simulink model "attitude_control"  (R2024b)
settings: Solver=FixedStepAuto  StartTime=0.0  StopTime=1000  FixedStep=1  RelTol=1e-3
values from neighbouring files (symbols this model uses):
  H0 = [30; 30; 30]    [initialcondition.m]
  I = [1759 0 0; 0 2758 0; 0 0 2171]    [initialcondition.m]
  kxd = 395.4913    [initialcondition.m]    (also in pd_fitness.m = x(4); pd_show.m = out.kxd)
  kxp = 18.1115    [initialcondition.m]    (also in pd_fitness.m = x(1); pd_show.m = out.kxp)
  kyd = 172.6452    [initialcondition.m]    (also in pd_fitness.m = x(5); pd_show.m = out.kyd)
  kyp = 7.3074    [initialcondition.m]    (also in pd_fitness.m = x(2); pd_show.m = out.kyp)
  kzd = 636.1855    [initialcondition.m]    (also in pd_fitness.m = x(6); pd_show.m = out.kzd)
  kzp = 21.1317    [initialcondition.m]    (also in pd_fitness.m = x(3); pd_show.m = out.kzp)
  qZYX = eul2quat(Euler0)    [initialcondition.m]
  w0 = [0; 0; 0]    [initialcondition.m]
settings Model: Creator=ThinkBook  LastModifiedBy=Lzy18
settings DebuggingCC: UnconnectedInputMsg=warning  UnconnectedOutputMsg=warning  UnconnectedLineMsg=warning
settings ModelReferenceCC: EnableRefExpFcnMdlSchedulingChecks=on
settings RTWCC: GPUComputeCapability=3.5  DLArmComputeVersion=19.05

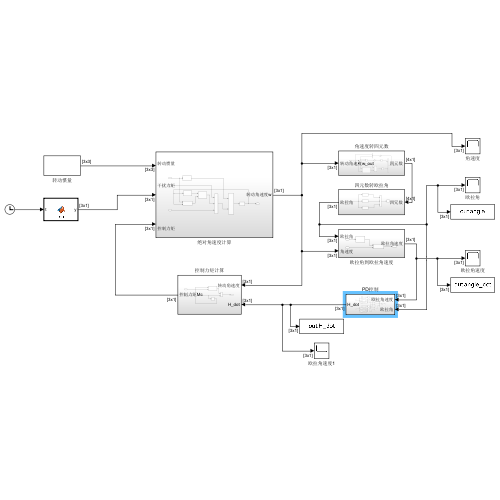
[thumbnail: Simulink's stored preview of the top-level diagram]
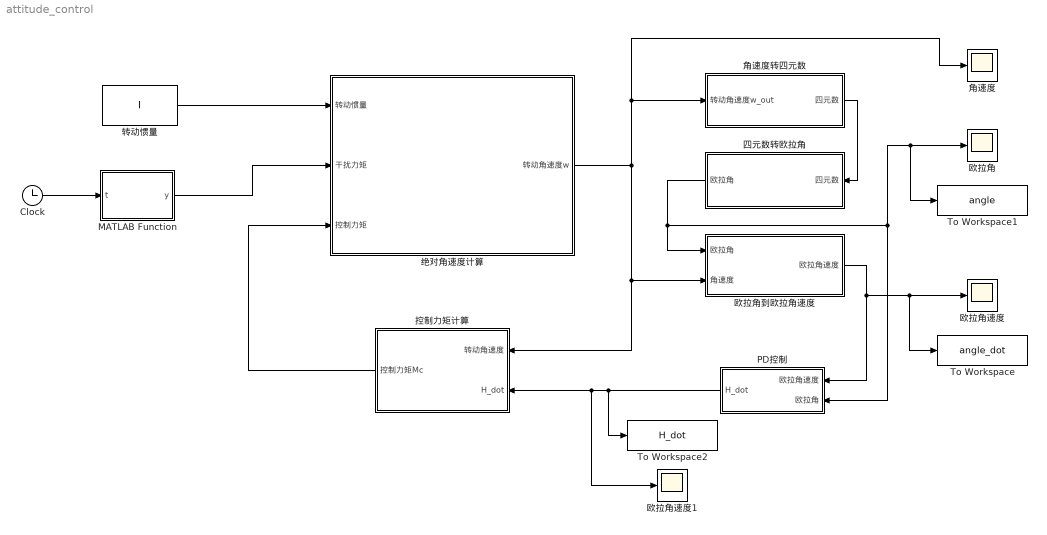
== system attitude_control ==
  Clock : Clock
  MATLAB Function : MATLAB Function  TreatAsAtomicUnit=on
  PD控制 : Subsystem
  To Workspace : ToWorkspace  VariableName=angle_dot  SampleTime=-1
  To Workspace1 : ToWorkspace  VariableName=angle  SampleTime=-1
  To Workspace2 : ToWorkspace  VariableName=H_dot  SampleTime=-1
  四元数转欧拉角 : Subsystem
  控制力矩计算 : Subsystem
  欧拉角 : Scope
  欧拉角到欧拉角速度 : Subsystem
  欧拉角速度 : Scope
  欧拉角速度1 : Scope
  绝对角速度计算 : Subsystem
  角速度 : Scope
  角速度转四元数 : Subsystem
  转动惯量 : Constant  Value=I
  wires:
  转动惯量/1 -> 绝对角速度计算/1(转动惯量)
  控制力矩计算/1(控制力矩Mc) -> 绝对角速度计算/3(控制力矩)
  绝对角速度计算/1(转动角速度w) -> 角速度/1, 角速度转四元数/1(转动角速度w_out), 控制力矩计算/1(转动角速度), 欧拉角到欧拉角速度/2(角速度)
  角速度转四元数/1(四元数) -> 四元数转欧拉角/1(四元数)
  PD控制/1(H_dot) -> To Workspace2/1, 欧拉角速度1/1, 控制力矩计算/2(H_dot)
  四元数转欧拉角/1(欧拉角) -> 欧拉角到欧拉角速度/1(欧拉角), PD控制/2(欧拉角), To Workspace1/1, 欧拉角/1
  MATLAB Function/1(y) -> 绝对角速度计算/2(干扰力矩)
  Clock/1 -> MATLAB Function/1(t)
  欧拉角到欧拉角速度/1(欧拉角速度) -> PD控制/1(欧拉角速度), To Workspace/1, 欧拉角速度/1

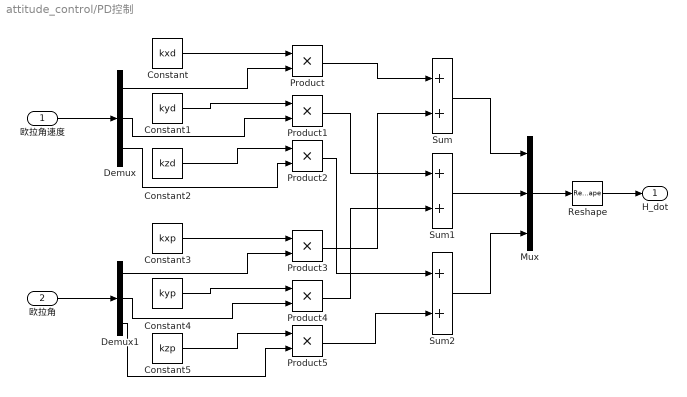
== system attitude_control/PD控制 ==
  欧拉角速度 : Inport
  欧拉角 : Inport  Port=2
  Constant : Constant  Value=kxd
  Constant1 : Constant  Value=kyd
  Constant2 : Constant  Value=kzd
  Constant3 : Constant  Value=kxp
  Constant4 : Constant  Value=kyp
  Constant5 : Constant  Value=kzp
  Demux : Demux  Outputs=3
  Demux1 : Demux  Outputs=3
  Mux : Mux  Inputs=3
  Product{,1..5} (6 alike) : Product
  Reshape : Reshape  OutputDimensionality=Customize  OutputDimensions=[3,1]
  Sum : Sum
  Sum1 : Sum
  Sum2 : Sum
  H_dot : Outport
  wires:
  欧拉角速度/1 -> Demux/1
  欧拉角/1 -> Demux1/1
  Demux/1 -> Product/2
  Constant/1 -> Product/1
  Constant1/1 -> Product1/1
  Demux/2 -> Product1/2
  Constant2/1 -> Product2/1
  Demux/3 -> Product2/2
  Constant5/1 -> Product5/1
  Constant3/1 -> Product3/1
  Demux1/1 -> Product3/2
  Constant4/1 -> Product4/1
  Demux1/2 -> Product4/2
  Demux1/3 -> Product5/2
  Product/1 -> Sum/1
  Product3/1 -> Sum/2
  Sum/1 -> Mux/1
  Sum1/1 -> Mux/2
  Sum2/1 -> Mux/3
  Product1/1 -> Sum1/1
  Product4/1 -> Sum1/2
  Product2/1 -> Sum2/1
  Product5/1 -> Sum2/2
  Mux/1 -> Reshape/1
  Reshape/1 -> H_dot/1

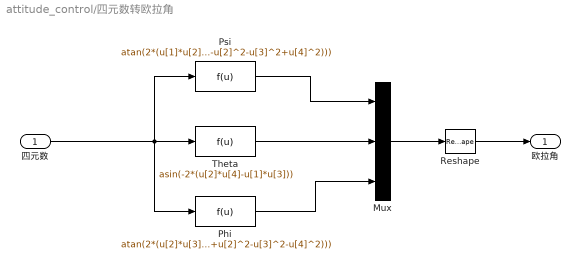
== system attitude_control/四元数转欧拉角 ==
  四元数 : Inport
  Mux : Mux  Inputs=3
  Phi : Fcn  Expr=atan(2*(u[2]*u[3]+u[1]*u[4]/(u[1]^2+u[2]^2-u[3]^2-u[4]^2)))
  Psi : Fcn  Expr=atan(2*(u[1]*u[2]+u[3]*u[4]/(u[1]^2-u[2]^2-u[3]^2+u[4]^2)))
  Reshape : Reshape  OutputDimensionality=Customize  OutputDimensions=[3,1]
  Theta : Fcn  Expr=asin(-2*(u[2]*u[4]-u[1]*u[3]))
  欧拉角 : Outport
  wires:
  Psi/1 -> Mux/1
  四元数/1 -> Phi/1, Psi/1, Theta/1
  Theta/1 -> Mux/2
  Phi/1 -> Mux/3
  Mux/1 -> Reshape/1
  Reshape/1 -> 欧拉角/1

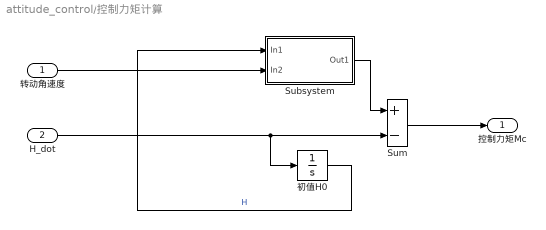
== system attitude_control/控制力矩计算 ==
  转动角速度 : Inport
  H_dot : Inport  Port=2
  Subsystem : Subsystem
      mask Display:
      | disp('Cross \nProduct')
      | port_label('input',1,'X')
      | port_label('input',2,'Y')
      | port_label('output',1,'X*Y')
  Sum : Sum  Inputs=+-
  初值H0 : Integrator  InitialCondition=H0
  控制力矩Mc : Outport
  wires:
  Sum/1 -> 控制力矩Mc/1
  转动角速度/1 -> Subsystem/2(In2)
  H_dot/1 -> Sum/2, 初值H0/1
  Subsystem/1(Out1) -> Sum/1
  初值H0/1 -> Subsystem/1(In1)  "H"

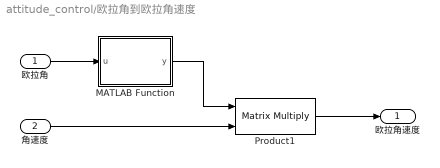
== system attitude_control/欧拉角到欧拉角速度 ==
  欧拉角 : Inport
  角速度 : Inport  Port=2
  MATLAB Function : MATLAB Function  TreatAsAtomicUnit=on
  Product1 : Product  Multiplication=Matrix(*)
  欧拉角速度 : Outport
  wires:
  Product1/1 -> 欧拉角速度/1
  欧拉角/1 -> MATLAB Function/1(u)
  MATLAB Function/1(y) -> Product1/1
  角速度/1 -> Product1/2

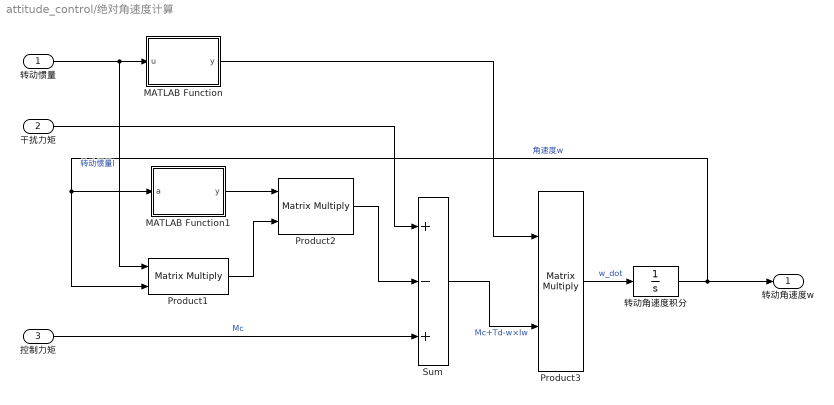
== system attitude_control/绝对角速度计算 ==
  转动惯量 : Inport
  干扰力矩 : Inport  Port=2
  控制力矩 : Inport  Port=3
  MATLAB Function : MATLAB Function  TreatAsAtomicUnit=on
  MATLAB Function1 : MATLAB Function  TreatAsAtomicUnit=on
  Product1 : Product  Multiplication=Matrix(*)
  Product2 : Product  Multiplication=Matrix(*)
  Product3 : Product  Multiplication=Matrix(*)
  Sum : Sum  Inputs=+-+
  转动角速度积分 : Integrator  InitialCondition=w0
  转动角速度w : Outport
  wires:
  Sum/1 -> Product3/2  "Mc+Td-w×Iw"
  Product3/1 -> 转动角速度积分/1  "w_dot"
  转动角速度积分/1 -> Product1/2, MATLAB Function1/1(a), 转动角速度w/1  "角速度w"
  转动惯量/1 -> MATLAB Function/1(u), Product1/1  "转动惯量I"
  控制力矩/1 -> Sum/3  "Mc"
  MATLAB Function/1(y) -> Product3/1
  MATLAB Function1/1(y) -> Product2/1
  Product1/1 -> Product2/2
  Product2/1 -> Sum/2
  干扰力矩/1 -> Sum/1

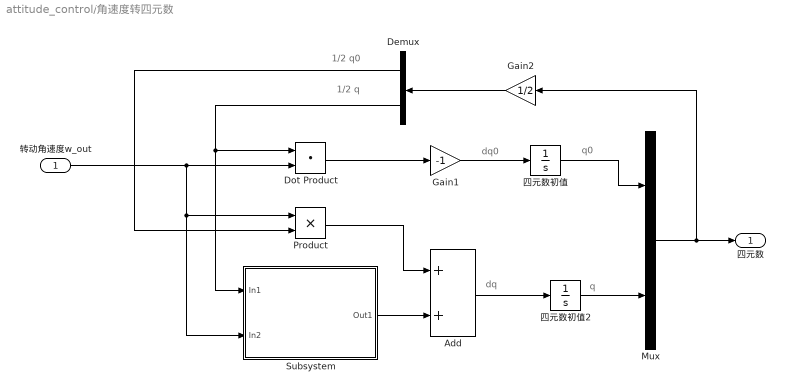
== system attitude_control/角速度转四元数 ==
  note: q
  note: dq
  note: dq0
  note: q0
  note: 1/2 q0
  note: 1/2 q
  转动角速度w_out : Inport
  Add : Sum
  Demux : Demux  Outputs=2
  Dot Product : DotProduct  OutDataTypeStr=Inherit: Inherit via internal rule
  Gain1 : Gain  Gain=-1
  Gain2 : Gain  Gain=1/2
  Mux : Mux  Inputs=[1 3]
  Product : Product
  Subsystem : Subsystem
      mask Display:
      | disp('Cross \nProduct')
      | port_label('input',1,'X')
      | port_label('input',2,'Y')
      | port_label('output',1,'X*Y')
  四元数初值 : Integrator  InitialCondition=qZYX(1)
  四元数初值2 : Integrator  InitialCondition=qZYX(2:4)'
  四元数 : Outport
  wires:
  Demux/2 -> Dot Product/1, Subsystem/1(In1)
  Gain1/1 -> 四元数初值/1
  Subsystem/1(Out1) -> Add/2
  四元数初值/1 -> Mux/1
  Demux/1 -> Product/2
  Gain2/1 -> Demux/1
  Mux/1 -> Gain2/1, 四元数/1
  转动角速度w_out/1 -> Product/1, Subsystem/2(In2), Dot Product/2
  Add/1 -> 四元数初值2/1
  Dot Product/1 -> Gain1/1
  四元数初值2/1 -> Mux/2
  Product/1 -> Add/1

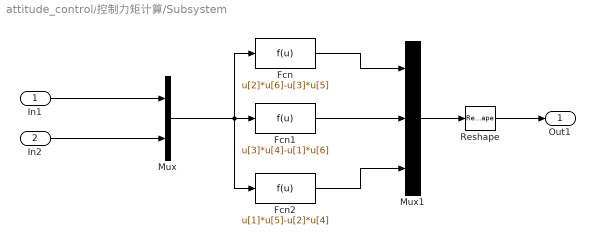
== system attitude_control/控制力矩计算/Subsystem ==
  In1 : Inport
  In2 : Inport  Port=2
  Fcn : Fcn  Expr=u[2]*u[6]-u[3]*u[5]
  Fcn1 : Fcn  Expr=u[3]*u[4]-u[1]*u[6]
  Fcn2 : Fcn  Expr=u[1]*u[5]-u[2]*u[4]
  Mux : Mux  Inputs=2
  Mux1 : Mux  Inputs=3
  Reshape : Reshape  OutputDimensionality=Customize  OutputDimensions=[3,1]
  Out1 : Outport
  wires:
  In2/1 -> Mux/2
  In1/1 -> Mux/1
  Fcn/1 -> Mux1/1
  Fcn1/1 -> Mux1/2
  Fcn2/1 -> Mux1/3
  Mux/1 -> Fcn2/1, Fcn/1, Fcn1/1
  Reshape/1 -> Out1/1
  Mux1/1 -> Reshape/1

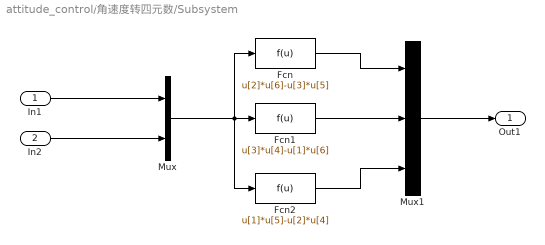
== system attitude_control/角速度转四元数/Subsystem ==
  In1 : Inport
  In2 : Inport  Port=2
  Fcn : Fcn  Expr=u[2]*u[6]-u[3]*u[5]
  Fcn1 : Fcn  Expr=u[3]*u[4]-u[1]*u[6]
  Fcn2 : Fcn  Expr=u[1]*u[5]-u[2]*u[4]
  Mux : Mux  Inputs=2
  Mux1 : Mux  Inputs=3
  Out1 : Outport
  wires:
  In2/1 -> Mux/2
  In1/1 -> Mux/1
  Fcn/1 -> Mux1/1
  Fcn1/1 -> Mux1/2
  Fcn2/1 -> Mux1/3
  Mux/1 -> Fcn2/1, Fcn/1, Fcn1/1
  Mux1/1 -> Out1/1

== matlab function attitude_control/绝对角速度计算/MATLAB Function ==
  data: u input; y output
function y = fcn(u)

y = inv(u);

end

== matlab function attitude_control/绝对角速度计算/MATLAB Function1 ==
  data: a input; y output
function y = fcn(a)
% Convert input vectors to 3x3 matrices
A=[0 -a(3) a(2);a(3) 0 -a(1);-a(2) a(1) 0];
% Calculate cross product of matrices
y=A;
end

== matlab function attitude_control/MATLAB Function ==
  data: t input; y output
function y = fcn(t)
w = 3;
y = [1*sin(w*t);
     2*cos(w*t+pi/3); 
     3*cos(w*t)];
end

== matlab function attitude_control/欧拉角到欧拉角速度/MATLAB Function ==
  data: u input; y output
function y = fcn(u)
Psi = u(1);
Theta = u(2);

y = [1 sin(Psi)*tan(Theta) cos(Psi)*tan(Theta);
    0 cos(Psi) -sin(Psi);
    0 sin(Psi)/cos(Theta) cos(Psi)/cos(Theta)];

end
